simulink library "Plant"  (R2024b)
settings: Solver=VariableStepAuto  StartTime=0.0  StopTime=10.0  RelTol=1e-3
undefined symbols (not defined in the file): slPart

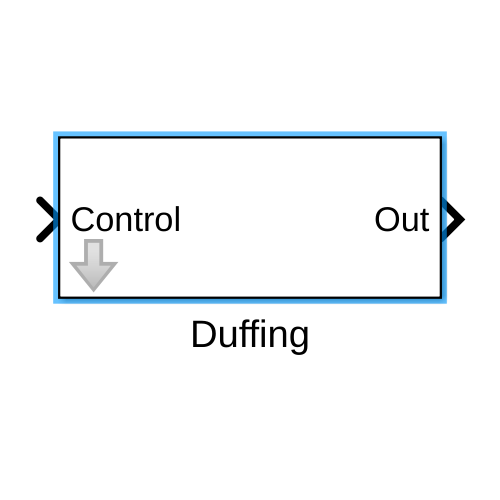
[thumbnail: Simulink's stored preview of the top-level diagram]
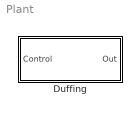
== system Plant ==
  Duffing : Subsystem  mask(slPart){obj=slPart}
      mask prompts: obj "slPart Object:"
      mask help: Container block for all slPart blocks
      mask init:
      | obj.maskInit(gcb);

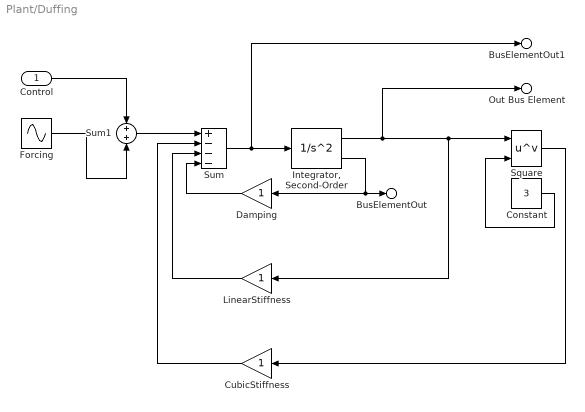
== system Plant/Duffing ==
  Control : Inport
  Constant : Constant  Value=3
  CubicStiffness : Gain
  Damping : Gain
  Forcing : Sin  SampleTime=0
  "Integrator, Second-Order" : SecondOrderIntegrator
  LinearStiffness : Gain
  Square : Math  Operator=pow
  Sum : Sum  Inputs=+---
  Sum1 : Sum
  Out Bus Element : Outport  PortName=Out  Element=x
  BusElementOut : Outport  PortName=Out  Element=v
  BusElementOut1 : Outport  PortName=Out  Element=a
  wires:
  Constant/1 -> Square/2
  Sum/1 -> BusElementOut1/1, "Integrator, Second-Order"/1
  Square/1 -> CubicStiffness/1
  "Integrator, Second-Order"/2 -> BusElementOut/1, Damping/1
  CubicStiffness/1 -> Sum/2
  Damping/1 -> Sum/4
  "Integrator, Second-Order"/1 -> Out Bus Element/1, LinearStiffness/1, Square/1
  LinearStiffness/1 -> Sum/3
  Forcing/1 -> Sum1/2
  Control/1 -> Sum1/1
  Sum1/1 -> Sum/1
